simulink model "InterfaceI2CDAC"  (R2016b)
settings: Solver=FixedStepAuto  StartTime=0.0  StopTime=inf  FixedStep=0.1  RelTol=1e-3  EnableMultiTasking=on
libraries: EEE481Arduino x3
settings Model: ExtModeTrigDuration=2  Creator=rsjoshi1  LastModifiedBy=rsjoshi1
settings OptimizationCC: LifeSpan=1  MaxStackSize=64
settings DebuggingCC: SFUnexpectedBacktrackingDiag=warning  SFNoUnconditionalDefaultTransitionDiag=warning  SFExecutionAtInitializationDiag=none
settings HardwareCC: ProdBitPerPointer=32  ProdBitPerSizeT=32  ProdBitPerPtrDiffT=32  ProdLargestAtomicInteger=Long  ProdLargestAtomicFloat=Double  ProdWordSize=32  ProdHWDeviceType=ARM Compatible->ARM Cortex
settings RTWCC: SystemTargetFile=ert.tlc  HardwareBoard=Arduino Due  TLCOptions=-aInlineSetEventsForThisBaseRateFcn=TLC_FALSE -aSuppressMultiTaskScheduler=TLC_FALSE -aRateBasedStepFcn=1  TemplateMakefile=ert_default_tmf  Description=Embedded Coder  GenerateReport=on  Toolchain=Arduino ARM v1.6.7  BuildConfiguration=Faster Runs  IncludeHyperlinkInReport=on  LaunchReport=on  GenerateTraceInfo=on  GenerateTraceReport=on  GenerateTraceReportSl=on  GenerateTraceReportSf=on  GenerateTraceReportEml=on
settings CodeAppCC: ForceParamTrailComments=on  IgnoreCustomStorageClasses=off  OperatorAnnotations=on  SimulinkDataObjDesc=on  SFDataObjDesc=on  MATLABFcnDesc=on  InsertBlockDesc=on  MATLABSourceComments=on
settings ERTTargetCC: SupportContinuousTime=on  SupportVariableSizeSignals=on
settings ConfigComp: CovMetricSettings=dw  CovHtmlReporting=on  CovSaveCumulativeToWorkspaceVar=on  CovSaveSingleToWorkspaceVar=on  CovExternalEMLEnable=off

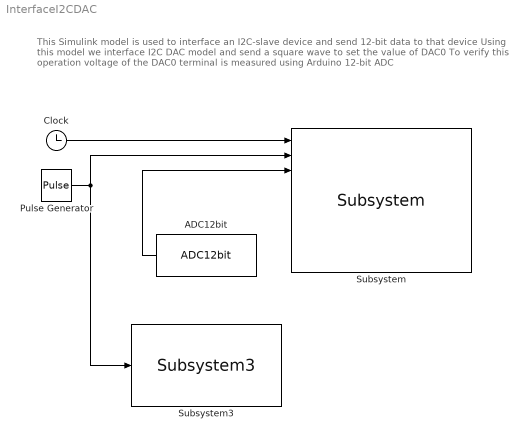
== system InterfaceI2CDAC ==
  note: This Simulink model is used to interface an I2C-slave device and send 12-bit data to that device
      | Using this model we interface I2C DAC model and send a square wave to set the value of DAC0
      | To verify this operation voltage of the DAC0 terminal is measured using Arduino 12-bit ADC
  ADC12bit : EEE481Arduino/ADC12bit  pinNum=5  Tsa=-1
  Clock : Clock
  Pulse Generator : DiscretePulseGenerator  PulseType=Time based  Amplitude=4000  Period=10  PulseWidth=5
  Subsystem : EEE481Arduino/Subsystem  Tsa=1  rate=0  per=0
  Subsystem3 : EEE481Arduino/Subsystem3  Tsa=Tsa  SlaveAdd=41
  wires:
  Pulse Generator/1 -> Subsystem/2, Subsystem3/1
  Clock/1 -> Subsystem/1
  ADC12bit/1 -> Subsystem/3
